simulink model "Eindaemmungsstrategien"  (R2020b)
settings: Solver=VariableStepAuto  StartTime=0.0  StopTime=100  RelTol=1e-3
model workspace (MAT data in the model file):
  I_strategie = 1
  i = 0.001
  k = 0.1
  r_strategie = 0
  s = Simulink.Parameter
  s.Value = 4
  s.DataType = 'auto'
  s.Dimensions = [1 1]
  tk = 0
  y0 = 0.01
libraries: simulink x1
settings Model: Creator=ypz  LastModifiedBy=ypz

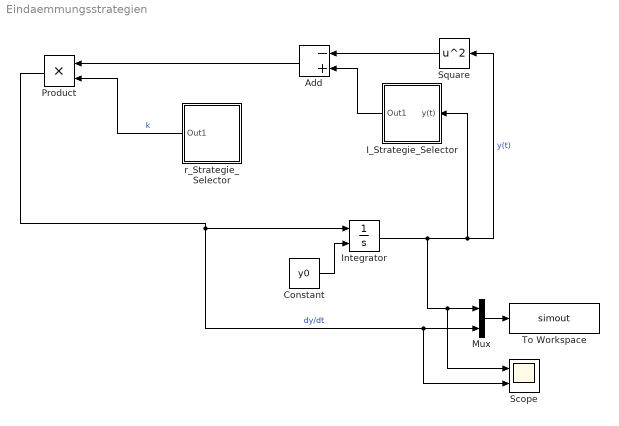
== system Eindaemmungsstrategien ==
  Add : Sum  Inputs=-+
  Constant : Constant  Value=y0
  I_Strategie_Selector : Subsystem
  Integrator : Integrator  InitialConditionSource=external
  Mux : Mux  Inputs=2
  Product : Product
  Scope : Scope  NumInputPorts=2
  Square : Math  Operator=square  SaturateOnIntegerOverflow=on
  To Workspace : ToWorkspace  VariableName=simout  SaveFormat=Timeseries  SampleTime=-1
  r_Strategie_Selector : Subsystem
  wires:
  Integrator/1 -> I_Strategie_Selector/1(y(t)), Square/1, Scope/1, Mux/1  "y(t)"
  Constant/1 -> Integrator/2
  Square/1 -> Add/1
  Add/1 -> Product/1
  Product/1 -> Integrator/1, Scope/2, Mux/2  "dy/dt"
  Mux/1 -> To Workspace/1
  r_Strategie_Selector/1(Out1) -> Product/2  "k"
  I_Strategie_Selector/1(Out1) -> Add/2

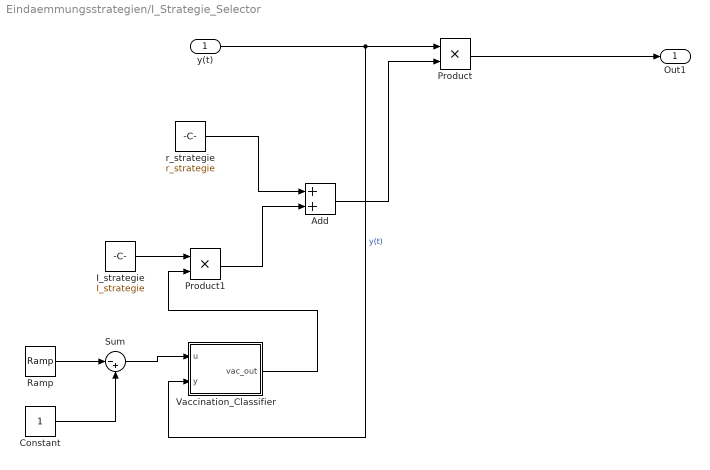
== system Eindaemmungsstrategien/I_Strategie_Selector ==
  y(t) : Inport
  Add : Sum
  Constant : Constant
  I_strategie : Constant  Value=I_strategie
  Product : Product
  Product1 : Product
  Ramp : simulink/Sources/Ramp  slope=i  start=0  InitialOutput=0
  Sum : Sum  Inputs=|-+
  Vaccination_Classifier : MATLAB Function  TreatAsAtomicUnit=on
  r_strategie : Constant  Value=r_strategie
  Out1 : Outport
  wires:
  y(t)/1 -> Vaccination_Classifier/2(y), Product/1  "y(t)"
  Product/1 -> Out1/1
  Add/1 -> Product/2
  r_strategie/1 -> Add/1
  I_strategie/1 -> Product1/1
  Product1/1 -> Add/2
  Ramp/1 -> Sum/1
  Constant/1 -> Sum/2
  Sum/1 -> Vaccination_Classifier/1(u)
  Vaccination_Classifier/1(vac_out) -> Product1/2

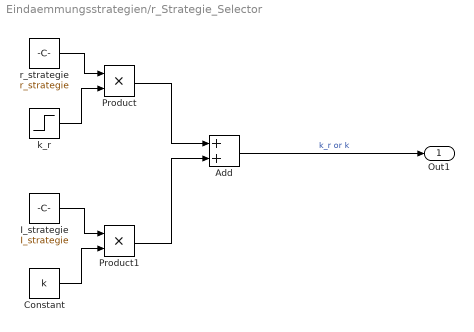
== system Eindaemmungsstrategien/r_Strategie_Selector ==
  Add : Sum
  Constant : Constant  Value=k
  I_strategie : Constant  Value=I_strategie
  Product : Product
  Product1 : Product
  k_r : Step  Time=tk  Before=k  After=k/3  SampleTime=0
  r_strategie : Constant  Value=r_strategie
  Out1 : Outport
  wires:
  Add/1 -> Out1/1  "k_r or k"
  r_strategie/1 -> Product/1
  k_r/1 -> Product/2
  I_strategie/1 -> Product1/1
  Constant/1 -> Product1/2
  Product/1 -> Add/1
  Product1/1 -> Add/2

== matlab function Eindaemmungsstrategien/I_Strategie_Selector/Vaccination_Classifier ==
  data: u input; vac_out output; y input
function vac_out = fcn(u,y)
% Im SI Modell muss angenommen werden, dass Infizierte nicht mehr geimpft
% werden können. Somit ergibt sich, i*t <= 1-y. u steht hier für 1-i*t
if u >= y
    vac_out = u;
else
    % Alle gesunde Menschen sind schon geimpft. Weitere infektionen sind
    % somit ausgeschlossen. y = const.
    vac_out = y;
end
